simulink model "Q1A"  (R2017b)
settings: Solver=VariableStepAuto  StartTime=0.0  StopTime=100000  RelTol=1e-3  EnableMultiTasking=on
undefined symbols (not defined in the file): m, n
settings Model: Creator=The MathWorks, Inc.  LastModifiedBy=Siamak
settings DataIOCC: LimitDataPoints=on  SaveFormat=Array
settings OptimizationCC: LifeSpan=inf
settings DebuggingCC: AllowSymbolicDim=off  SFUnexpectedBacktrackingDiag=warning  SFNoUnconditionalDefaultTransitionDiag=warning  SFExecutionAtInitializationDiag=none
settings ModelReferenceCC: PropagateSignalLabelsOutOfModel=off
settings CodeAppCC: StateflowObjectComments=on
settings GRTTargetCC: TargetLangStandard=C89/C90 (ANSI)  GeneratePreprocessorConditionals=Disable all
settings ConfigComp: CovMetricSettings=dw  CovHtmlReporting=on  CovSaveCumulativeToWorkspaceVar=on  CovSaveSingleToWorkspaceVar=on  CovExternalEMLEnable=off  CovSFcnEnable=off

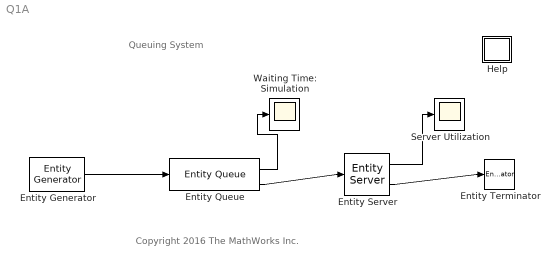
== system Q1A ==
  note: Copyright 2016 The MathWorks Inc.
  note: Queuing System
  Entity Generator : EntityGenerator  OutputPortMessageModes=m  IntergenerationTimeAction=dt = exponentialArrivalTime();  EntityType=Structured  EntityTypeName=Entity
  Entity Queue : EntityQueue  InputPortMessageModes=m  OutputPortMessageModes=n,m  Capacity=Inf  AverageWait=on
      settings: OutputPortMap=o2,o5
  Entity Server : EntityServer  InputPortMessageModes=m  OutputPortMessageModes=n,m  Capacity=1  ServiceTimeSource=MATLAB action  ServiceTimeAction=|  Utilization=on
      | % Exponential service time with rate 1
      | mean = 1;
      | dt   = -mean * log(1 - rand());
      settings: OutputPortMap=o5,o9
  Entity Terminator : EntityTerminator  InputPortMessageModes=m
  Help : Subsystem
      settings: OpenFcn=showdemo(bdroot(gcb));
      mask Display: disp('?')
  Server Utilization : Scope
  Waiting Time: Simulation : Scope
  wires:
  Entity Generator/1 -> Entity Queue/1
  Entity Queue/2 -> Entity Server/1
  Entity Server/2 -> Entity Terminator/1
  Entity Queue/1 -> Waiting Time: Simulation/1
  Entity Server/1 -> Server Utilization/1

== system Q1A/Help ==
